simulink model "AL_Model"  (R2023b)
settings: Solver=VariableStepAuto  StartTime=0.0  StopTime=10.0  RelTol=1e-3
values from neighbouring files (symbols this model uses):
  beta = Kth    (= 0.0003)    [AL_parameters.m]    (also in set_params.m = 3.7343e-06)
  Dm = 0.00240    (= 0.0024)    [AL_parameters.m]    (also in beta_estimation.m)
  Dt = 0.167    [AL_parameters.m]    (also in beta_estimation.m)
  g = 9.81    [AL_parameters.m]    (also in beta_estimation.m)
  gamma = 0    [AL_parameters.m]    (also in fan.m = params(4))
  Jeq = Jr + Jh + Jprop    (= 4.40304e-05)    [AL_parameters.m]
  Jp = 0.0232    [AL_parameters.m]    (also in beta_estimation.m; set_params.m)
  Kcp = 0    [AL_parameters.m]
  kDp = 0    [AL_parameters.m]
  ke = kt    (= 0.042)    [AL_parameters.m]
  kFp = 0    [AL_parameters.m]
  kt = 4.20e-2    (= 0.042)    [AL_parameters.m]
  Mb = 1.07    [AL_parameters.m]    (also in beta_estimation.m)
  Rm = 8.40    (= 8.4)    [AL_parameters.m]
libraries: slpidlib x2
settings Model: Creator=HP  LastModifiedBy=franc

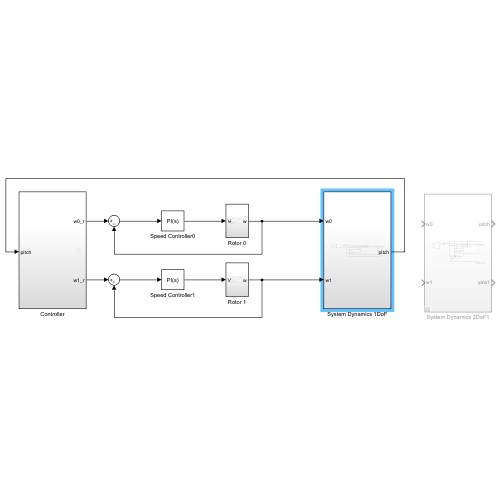
[thumbnail: Simulink's stored preview of the top-level diagram]
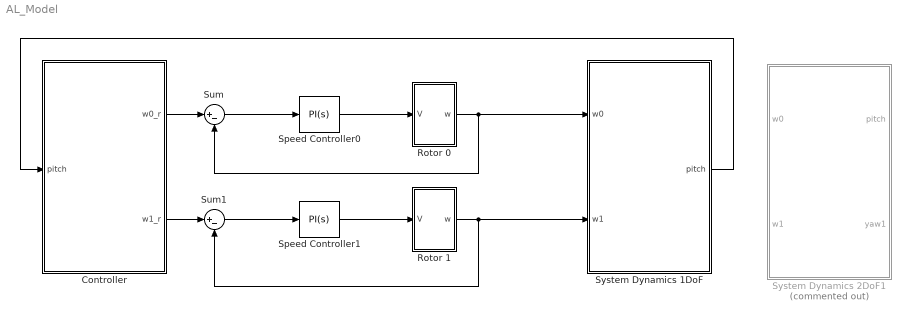
== system AL_Model ==
  Controller : Subsystem
  Rotor 0 : Subsystem
  Rotor 1 : Subsystem
  Speed Controller0 : slpidlib/PID Controller  Controller=PI  Form=Parallel  TimeDomain=Continuous-time  UseExternalTs=off  SampleTime=-1  IntegratorMethod=Forward Euler  FilterMethod=Forward Euler  ControllerParametersSource=internal  P=1  I=1  UseKiTs=off  D=0  N=100  UseFilter=on  TunerSelectOption=Transfer Function Based (PID Tuner App)  InitialConditionSource=internal  InitialConditionForIntegrator=0  InitialConditionForFilter=0  DifferentiatorICPrevScaledInput=0  ExternalReset=none  TrackingMode=off  Kt=1  LimitOutput=off  SatLimitsSource=internal  UpperSaturationLimit=inf  LowerSaturationLimit=-inf  LinearizeAsGain=on  AntiWindupMode=none  Kb=1  LimitIntegrator=off  UpperIntegratorSaturationLimit=inf  LowerIntegratorSaturationLimit=-inf  POutMin=[]  POutMax=[]  IOutMin=[]  IOutMax=[]  DOutMin=[]  DOutMax=[]  NOutMin=[]  NOutMax=[]  SumOutMin=[]  SumOutMax=[]  SaturationOutMin=[]  SaturationOutMax=[]  PParamMin=[]  PParamMax=[]  IParamMin=[]  IParamMax=[]  DParamMin=[]  DParamMax=[]  NParamMin=[]  NParamMax=[]  KbParamMin=[]  KbParamMax=[]  KtParamMin=[]  KtParamMax=[]  KbOutMin=[]  KbOutMax=[]  KtOutMin=[]  KtOutMax=[]  IntegratorOutMin=[]  IntegratorOutMax=[]  FilterOutMin=[]  FilterOutMax=[]  SumI1OutMin=[]  SumI1OutMax=[]  SumI2OutMin=[]  SumI2OutMax=[]  SumI3OutMin=[]  SumI3OutMax=[]  SumI4OutMin=[]  SumI4OutMax=[]  SumDOutMin=[]  SumDOutMax=[]  DifferentiatorOutMin=[]  DifferentiatorOutMax=[]  FilterDiffOutCoefMin=[]  FilterDiffOutCoefMax=[]  ReciprocalOutMin=[]  ReciprocalOutMax=[]  SumDenOutMin=[]  SumDenOutMax=[]  SumNumOutMin=[]  SumNumOutMax=[]  DivideOutMin=[]  DivideOutMax=[]  UdiffTsProdOutMin=[]  UdiffTsProdOutMax=[]  NTsProdOutMin=[]  NTsProdOutMax=[]  UintegralTsProdOutMin=[]  UintegralTsProdOutMax=[]  UngainTsProdOutMin=[]  UngainTsProdOutMax=[]  ClampingZeroOutDataTypeStr=Inherit: Inherit via back propagation  ClampingZeroOutMin=[]  ClampingZeroOutMax=[]  FilterDenConstantOutDataTypeStr=Inherit: Inherit via back propagation  FilterDenConstantOutMin=[]  FilterDenConstantOutMax=[]  PCopyOutDataTypeStr=Inherit: Inherit via back propagation  PCopyOutMin=[]  PCopyOutMax=[]  NCopyOutDataTypeStr=Inherit: Inherit via back propagation  NCopyOutMin=[]  NCopyOutMax=[]  IntegratorContinuousStateAttributes=''  IntegratorStateMustResolveToSignalObject=off  IntegratorRTWStateStorageClass=Auto  FilterContinuousStateAttributes=''  FilterStateMustResolveToSignalObject=off  FilterRTWStateStorageClass=Auto  ParallelPVariant=InternalParameters  IdealPVariant=Disabled  IVariant=InternalParameters  DVariant=Disabled  IntegratorVariant=Continuous  SatVariant=Disabled  AWVariant=Passthrough  PCopyVariant=Disabled  TRVariant=Disabled  FdbkBlocksVariant=Forward  IdealPFdbkVariant=Disabled  SatFdbkVariant=Disabled  DerivativeFilterVariant=Disabled  NVariant=Disabled  NCopyVariant=Disabled_SignalSpec  FilterICVariant=Disabled  IntegratorICVariant=InternalICs  ExternalResetVariant=Disabled  TRSumVariant=Passthrough  SumFdbkVariant=Disabled  SumVariant=Sum_PI  TsampFilterVariant=InternalTs  TsampNgainVariant=Passthrough  TsampIntegralVariant=Disabled_SignalSpec  ExternalSaturationOutDataTypeStr=Inherit: Same as second input
  Speed Controller1 : slpidlib/PID Controller  Controller=PI  Form=Parallel  TimeDomain=Continuous-time  UseExternalTs=off  SampleTime=-1  IntegratorMethod=Forward Euler  FilterMethod=Forward Euler  ControllerParametersSource=internal  P=1  I=1  UseKiTs=off  D=0  N=100  UseFilter=on  TunerSelectOption=Transfer Function Based (PID Tuner App)  InitialConditionSource=internal  InitialConditionForIntegrator=0  InitialConditionForFilter=0  DifferentiatorICPrevScaledInput=0  ExternalReset=none  TrackingMode=off  Kt=1  LimitOutput=off  SatLimitsSource=internal  UpperSaturationLimit=inf  LowerSaturationLimit=-inf  LinearizeAsGain=on  AntiWindupMode=none  Kb=1  LimitIntegrator=off  UpperIntegratorSaturationLimit=inf  LowerIntegratorSaturationLimit=-inf  POutMin=[]  POutMax=[]  IOutMin=[]  IOutMax=[]  DOutMin=[]  DOutMax=[]  NOutMin=[]  NOutMax=[]  SumOutMin=[]  SumOutMax=[]  SaturationOutMin=[]  SaturationOutMax=[]  PParamMin=[]  PParamMax=[]  IParamMin=[]  IParamMax=[]  DParamMin=[]  DParamMax=[]  NParamMin=[]  NParamMax=[]  KbParamMin=[]  KbParamMax=[]  KtParamMin=[]  KtParamMax=[]  KbOutMin=[]  KbOutMax=[]  KtOutMin=[]  KtOutMax=[]  IntegratorOutMin=[]  IntegratorOutMax=[]  FilterOutMin=[]  FilterOutMax=[]  SumI1OutMin=[]  SumI1OutMax=[]  SumI2OutMin=[]  SumI2OutMax=[]  SumI3OutMin=[]  SumI3OutMax=[]  SumI4OutMin=[]  SumI4OutMax=[]  SumDOutMin=[]  SumDOutMax=[]  DifferentiatorOutMin=[]  DifferentiatorOutMax=[]  FilterDiffOutCoefMin=[]  FilterDiffOutCoefMax=[]  ReciprocalOutMin=[]  ReciprocalOutMax=[]  SumDenOutMin=[]  SumDenOutMax=[]  SumNumOutMin=[]  SumNumOutMax=[]  DivideOutMin=[]  DivideOutMax=[]  UdiffTsProdOutMin=[]  UdiffTsProdOutMax=[]  NTsProdOutMin=[]  NTsProdOutMax=[]  UintegralTsProdOutMin=[]  UintegralTsProdOutMax=[]  UngainTsProdOutMin=[]  UngainTsProdOutMax=[]  ClampingZeroOutDataTypeStr=Inherit: Inherit via back propagation  ClampingZeroOutMin=[]  ClampingZeroOutMax=[]  FilterDenConstantOutDataTypeStr=Inherit: Inherit via back propagation  FilterDenConstantOutMin=[]  FilterDenConstantOutMax=[]  PCopyOutDataTypeStr=Inherit: Inherit via back propagation  PCopyOutMin=[]  PCopyOutMax=[]  NCopyOutDataTypeStr=Inherit: Inherit via back propagation  NCopyOutMin=[]  NCopyOutMax=[]  IntegratorContinuousStateAttributes=''  IntegratorStateMustResolveToSignalObject=off  IntegratorRTWStateStorageClass=Auto  FilterContinuousStateAttributes=''  FilterStateMustResolveToSignalObject=off  FilterRTWStateStorageClass=Auto  ParallelPVariant=InternalParameters  IdealPVariant=Disabled  IVariant=InternalParameters  DVariant=Disabled  IntegratorVariant=Continuous  SatVariant=Disabled  AWVariant=Passthrough  PCopyVariant=Disabled  TRVariant=Disabled  FdbkBlocksVariant=Forward  IdealPFdbkVariant=Disabled  SatFdbkVariant=Disabled  DerivativeFilterVariant=Disabled  NVariant=Disabled  NCopyVariant=Disabled_SignalSpec  FilterICVariant=Disabled  IntegratorICVariant=InternalICs  ExternalResetVariant=Disabled  TRSumVariant=Passthrough  SumFdbkVariant=Disabled  SumVariant=Sum_PI  TsampFilterVariant=InternalTs  TsampNgainVariant=Passthrough  TsampIntegralVariant=Disabled_SignalSpec  ExternalSaturationOutDataTypeStr=Inherit: Same as second input
  Sum : Sum  Inputs=|+-
  Sum1 : Sum  Inputs=|+-
  System Dynamics 1DoF : Subsystem
  System Dynamics 2DoF1 : Subsystem  Commented=on
  wires:
  Speed Controller0/1 -> Rotor 0/1(V)
  Speed Controller1/1 -> Rotor 1/1(V)
  Sum1/1 -> Speed Controller1/1
  Sum/1 -> Speed Controller0/1
  Rotor 0/1(w) -> Sum/2, System Dynamics 1DoF/1(w0)
  Rotor 1/1(w) -> Sum1/2, System Dynamics 1DoF/2(w1)
  Controller/1(w0_r) -> Sum/1
  Controller/2(w1_r) -> Sum1/1
  System Dynamics 1DoF/1(pitch) -> Controller/1(pitch)

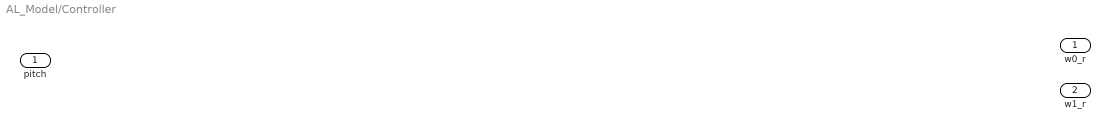
== system AL_Model/Controller ==
  pitch : Inport
  w0_r : Outport
  w1_r : Outport  Port=2

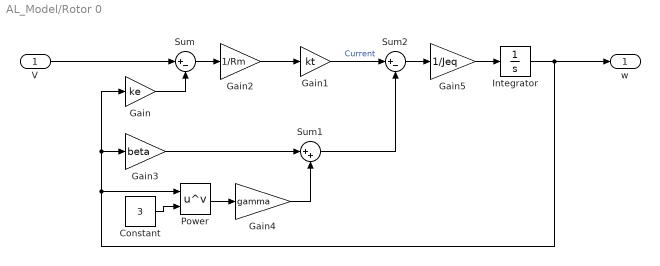
== system AL_Model/Rotor 0 ==
  V : Inport
  Constant : Constant  Value=3
  Gain : Gain  Gain=ke
  Gain1 : Gain  Gain=kt
  Gain2 : Gain  Gain=1/Rm
  Gain3 : Gain  Gain=beta
  Gain4 : Gain  Gain=gamma
  Gain5 : Gain  Gain=1/Jeq
  Integrator : Integrator
  Power : Math  Operator=pow
  Sum : Sum  Inputs=|+-
  Sum1 : Sum  Inputs=|++
  Sum2 : Sum  Inputs=|+-
  w : Outport
  wires:
  Gain3/1 -> Sum1/1
  V/1 -> Sum/1
  Gain1/1 -> Sum2/1  "Current"
  Power/1 -> Gain4/1
  Gain2/1 -> Gain1/1
  Gain/1 -> Sum/2
  Gain5/1 -> Integrator/1
  Sum1/1 -> Sum2/2
  Integrator/1 -> w/1, Power/1, Gain/1, Gain3/1
  Gain4/1 -> Sum1/2
  Sum/1 -> Gain2/1
  Sum2/1 -> Gain5/1
  Constant/1 -> Power/2

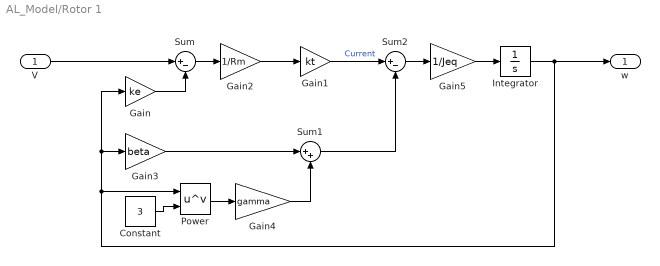
== system AL_Model/Rotor 1 ==
  V : Inport
  Constant : Constant  Value=3
  Gain : Gain  Gain=ke
  Gain1 : Gain  Gain=kt
  Gain2 : Gain  Gain=1/Rm
  Gain3 : Gain  Gain=beta
  Gain4 : Gain  Gain=gamma
  Gain5 : Gain  Gain=1/Jeq
  Integrator : Integrator
  Power : Math  Operator=pow
  Sum : Sum  Inputs=|+-
  Sum1 : Sum  Inputs=|++
  Sum2 : Sum  Inputs=|+-
  w : Outport
  wires:
  Gain3/1 -> Sum1/1
  V/1 -> Sum/1
  Gain1/1 -> Sum2/1  "Current"
  Power/1 -> Gain4/1
  Gain2/1 -> Gain1/1
  Gain/1 -> Sum/2
  Gain5/1 -> Integrator/1
  Sum1/1 -> Sum2/2
  Integrator/1 -> w/1, Power/1, Gain/1, Gain3/1
  Gain4/1 -> Sum1/2
  Sum/1 -> Gain2/1
  Sum2/1 -> Gain5/1
  Constant/1 -> Power/2

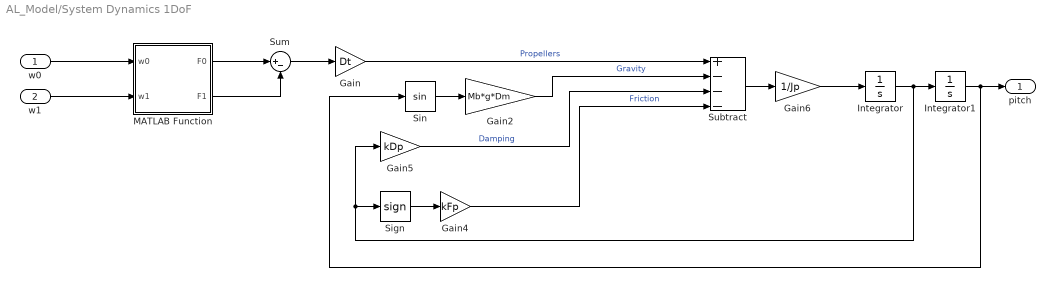
== system AL_Model/System Dynamics 1DoF ==
  w0 : Inport
  w1 : Inport  Port=2
  Gain : Gain  Gain=Dt
  Gain2 : Gain  Gain=Mb*g*Dm
  Gain4 : Gain  Gain=kFp
  Gain5 : Gain  Gain=kDp
  Gain6 : Gain  Gain=1/Jp
  Integrator : Integrator
  Integrator1 : Integrator
  MATLAB Function : MATLAB Function  TreatAsAtomicUnit=on
  Sign : Signum
  Sin : Trigonometry
  Subtract : Sum  Inputs=+---
  Sum : Sum  Inputs=|+-
  pitch : Outport
  wires:
  w0/1 -> MATLAB Function/1(w0)
  w1/1 -> MATLAB Function/2(w1)
  Integrator1/1 -> pitch/1, Sin/1
  Sin/1 -> Gain2/1
  MATLAB Function/2(F1) -> Sum/2
  Sum/1 -> Gain/1
  Gain2/1 -> Subtract/2  "Gravity"
  Sign/1 -> Gain4/1
  Integrator/1 -> Integrator1/1, Gain5/1, Sign/1
  Gain5/1 -> Subtract/3  "Damping"
  Gain4/1 -> Subtract/4  "Friction"
  Subtract/1 -> Gain6/1
  Gain6/1 -> Integrator/1
  Gain/1 -> Subtract/1  "Propellers"
  MATLAB Function/1(F0) -> Sum/1

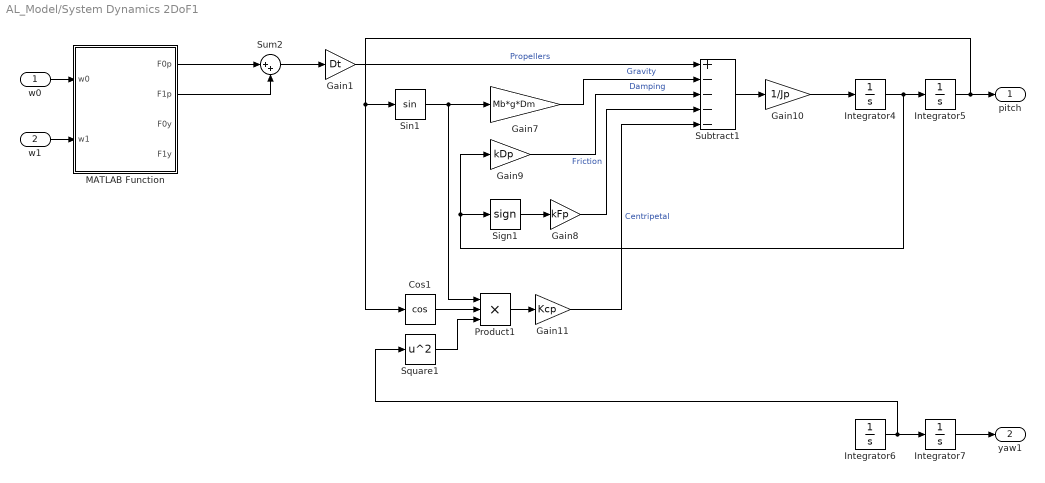
== system AL_Model/System Dynamics 2DoF1 ==
  w0 : Inport
  w1 : Inport  Port=2
  Cos1 : Trigonometry  Operator=cos
  Gain1 : Gain  Gain=Dt
  Gain10 : Gain  Gain=1/Jp
  Gain11 : Gain  Gain=Kcp
  Gain7 : Gain  Gain=Mb*g*Dm
  Gain8 : Gain  Gain=kFp
  Gain9 : Gain  Gain=kDp
  Integrator{4..7} (4 alike) : Integrator
  MATLAB Function : MATLAB Function  TreatAsAtomicUnit=on
  Product1 : Product  Inputs=3
  Sign1 : Signum
  Sin1 : Trigonometry
  Square1 : Math  Operator=square
  Subtract1 : Sum  Inputs=+----
  Sum2 : Sum  Inputs=|++
  pitch : Outport
  yaw1 : Outport  Port=2
  wires:
  w0/1 -> MATLAB Function/1(w0)
  w1/1 -> MATLAB Function/2(w1)
  Gain10/1 -> Integrator4/1
  Gain7/1 -> Subtract1/2  "Gravity"
  Gain8/1 -> Subtract1/4  "Friction"
  Gain1/1 -> Subtract1/1  "Propellers"
  Sum2/1 -> Gain1/1
  Subtract1/1 -> Gain10/1
  Sign1/1 -> Gain8/1
  Gain9/1 -> Subtract1/3  "Damping"
  Integrator5/1 -> pitch/1, Cos1/1, Sin1/1
  MATLAB Function/1(F0p) -> Sum2/1
  MATLAB Function/2(F1p) -> Sum2/2
  Integrator4/1 -> Integrator5/1, Gain9/1, Sign1/1
  Sin1/1 -> Product1/1, Gain7/1
  Square1/1 -> Product1/3
  Cos1/1 -> Product1/2
  Product1/1 -> Gain11/1
  Gain11/1 -> Subtract1/5  "Centripetal"
  Integrator7/1 -> yaw1/1
  Integrator6/1 -> Square1/1, Integrator7/1

== matlab function AL_Model/System Dynamics 2DoF1/MATLAB Function ==
  data: w0 input; F0p output; w1 input; F1p output; F0y output; F1y output
function [F0p,F1p,F0y,F1y] = fcn(w0, w1)
if w0>=0
    F0p = k0pp1*w0^2 + k0pp2*w0;
    F0y = k0yp1*w0^2 + k0yp2*w0;
else
    F0p = k0pn1*w0^2 + k0pn2*w0;
    F0y = k0yn1*w0^2 + k0yn2*w0;
end
if w1>=0
    F1p = k1pp1*w1^2 + k1pp2*w1;
    F1y = k1yp1*w1^2 + k1yp2*w1;
else
    F1p = k1pn1*w1^2 + k1pn2*w1;
    F1y = k1yn1*w1^2 + k1yn2*w1;
end

== matlab function AL_Model/System Dynamics 1DoF/MATLAB Function ==
  data: w0 input; F0 output; w1 input; F1 output
function [F0,F1] = fcn(w0, w1)
if w0>=0
    F0 = k0pp1*w0^2 + k0pp2*w0;
else
    F0 = k0pn1*w0^2 + k0pn2*w0;
end
if w1>=0
    F1 = k1pp1*w1^2 + k1pp2*w1;
else
    F1 = k1pn1*w1^2 + k1pn2*w1;
end
